simulink model "current_ctl_pi"  (R2023a)
settings: configuration reference "config" (kept outside this file)
model workspace (MAT data in the model file):
  bw = Simulink.Parameter
  bw.Value = 100
  bw.Description = '电流环百分比增益 %  100 表示 100%'
  bw.DataType = 'single'
  bw.Complexity = 'real'
  bw.Dimensions = [1 1]
  dt = Simulink.Parameter
  dt.Value = 5e-05
  dt.Description = '电流环运行频率 用于增益计算'
  dt.DataType = 'single'
  dt.Complexity = 'real'
  dt.Dimensions = [1 1]
  flux = Simulink.Parameter
  flux.Value = 0.0071333
  flux.Description = '磁链系数 Wb'
  flux.DataType = 'single'
  flux.Complexity = 'real'
  flux.Dimensions = [1 1]
  fs = Simulink.Parameter
  fs.Value = 20000
  fs.Description = '电流环运行频率 用于增益计算'
  fs.DataType = 'single'
  fs.Complexity = 'real'
  fs.Dimensions = [1 1]
  kFs = Simulink.Parameter
  kFs.Value = 20000
  kFs.Description = '电流环控制频率 HZ  用于设定模块仿真'
  kFs.DataType = 'double'
  kFs.Complexity = 'real'
  kFs.Dimensions = [1 1]
  ld = Simulink.Parameter
  ld.Value = 0.00059
  ld.Description = '定子电感 H'
  ld.DataType = 'single'
  ld.Complexity = 'real'
  ld.Dimensions = [1 1]
  ld_inv = Simulink.Parameter
  ld_inv.Value = 1694.91525424
  ld_inv.Description = '定子电感 H'
  ld_inv.DataType = 'single'
  ld_inv.Complexity = 'real'
  ld_inv.Dimensions = [1 1]
  lq = Simulink.Parameter
  lq.Value = 0.00059
  lq.Description = '定子电感 H'
  lq.DataType = 'single'
  lq.Complexity = 'real'
  lq.Dimensions = [1 1]
  lq_inv = Simulink.Parameter
  lq_inv.Value = 1694.91525424
  lq_inv.Description = '定子电感 H'
  lq_inv.DataType = 'single'
  lq_inv.Complexity = 'real'
  lq_inv.Dimensions = [1 1]
  r = Simulink.Parameter
  r.Value = 1.02
  r.Description = '定子电阻 ohm'
  r.DataType = 'single'
  r.Complexity = 'real'
  r.Dimensions = [1 1]
libraries: simulink x4, eeTransforms x2
settings Model: DataDictionary=model_config.sldd  ParameterArgumentNames=bw,dt,flux,fs,ld,ld_inv,lq,lq_inv,r  Creator=huangcheng  LastModifiedBy=Administrator
settings ConfigSetRef: SourceName=config

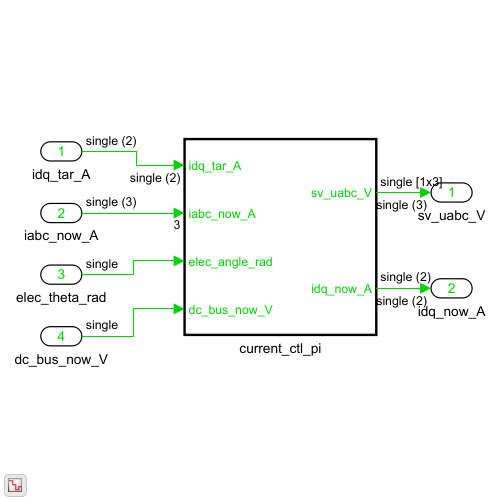
[thumbnail: Simulink's stored preview of the top-level diagram]
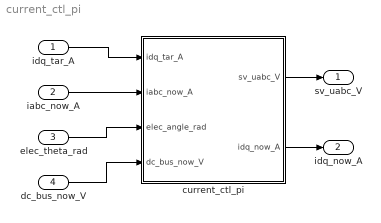
== system current_ctl_pi ==
  idq_tar_A : Inport  OutDataTypeStr=single  PortDimensions=2
  iabc_now_A : Inport  Port=2  OutDataTypeStr=single  PortDimensions=3
  elec_theta_rad : Inport  Port=3  OutDataTypeStr=single  PortDimensions=1
  dc_bus_now_V : Inport  Port=4
  current_ctl_pi : Subsystem  TreatAsAtomicUnit=on  SystemSampleTime=1/kFs
  sv_uabc_V : Outport  OutDataTypeStr=single  PortDimensions=3
  idq_now_A : Outport  Port=2  OutDataTypeStr=single  PortDimensions=2
  wires:
  current_ctl_pi/1(sv_uabc_V) -> sv_uabc_V/1
  idq_tar_A/1 -> current_ctl_pi/1(idq_tar_A)
  elec_theta_rad/1 -> current_ctl_pi/3(elec_angle_rad)
  iabc_now_A/1 -> current_ctl_pi/2(iabc_now_A)
  current_ctl_pi/2(idq_now_A) -> idq_now_A/1
  dc_bus_now_V/1 -> current_ctl_pi/4(dc_bus_now_V)

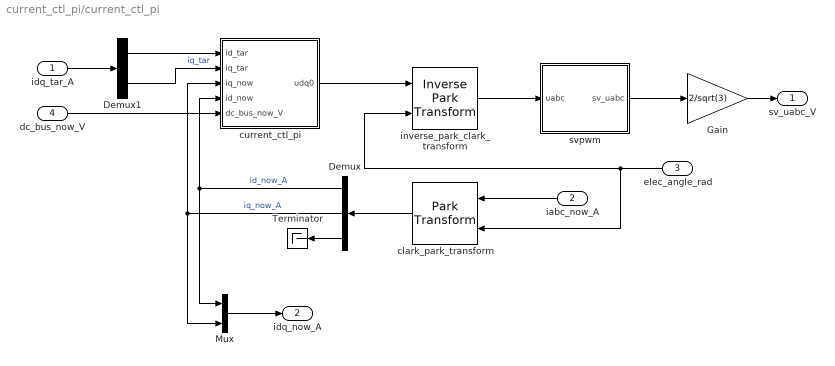
== system current_ctl_pi/current_ctl_pi ==
  idq_tar_A : Inport  OutDataTypeStr=single  PortDimensions=2
  iabc_now_A : Inport  Port=2  PortDimensions=3
  elec_angle_rad : Inport  Port=3
  dc_bus_now_V : Inport  Port=4
  Demux : Demux  Outputs=3
  Demux1 : Demux  Outputs=2
  Gain : Gain  Gain=2/sqrt(3)
  Mux : Mux  Inputs=2
  Terminator : Terminator
  "clark_park_transform " : eeTransforms/Park Transform  AxisAlignment=D-axis  PowerInvariant=off
  current_ctl_pi : Subsystem  SystemSampleTime=5e-5
  inverse_park_clark_transform : eeTransforms/Inverse Park Transform  AxisAlignment=D-axis  PowerInvariant=off
      settings: LibrarySourceBlock=|
      | ee_sl_lib/Mathematical
      | Transforms/Inverse
      | Park Transform
  "svpwm " : MATLAB Function
  sv_uabc_V : Outport
  idq_now_A : Outport  Port=2
  wires:
  "clark_park_transform "/1 -> Demux/1
  Demux/2 -> Mux/2, current_ctl_pi/3(iq_now)  "iq_now_A"
  Demux1/2 -> current_ctl_pi/2(iq_tar)  "iq_tar"
  idq_tar_A/1 -> Demux1/1
  elec_angle_rad/1 -> "clark_park_transform "/2, inverse_park_clark_transform/2
  inverse_park_clark_transform/1 -> "svpwm "/1(uabc)
  current_ctl_pi/1(udq0) -> inverse_park_clark_transform/1
  Demux/1 -> Mux/1, current_ctl_pi/4(id_now)  "id_now_A"
  Demux1/1 -> current_ctl_pi/1(id_tar)
  "svpwm "/1(sv_uabc) -> Gain/1
  iabc_now_A/1 -> "clark_park_transform "/1
  Demux/3 -> Terminator/1
  Mux/1 -> idq_now_A/1
  dc_bus_now_V/1 -> current_ctl_pi/5(dc_bus_now_V)
  Gain/1 -> sv_uabc_V/1

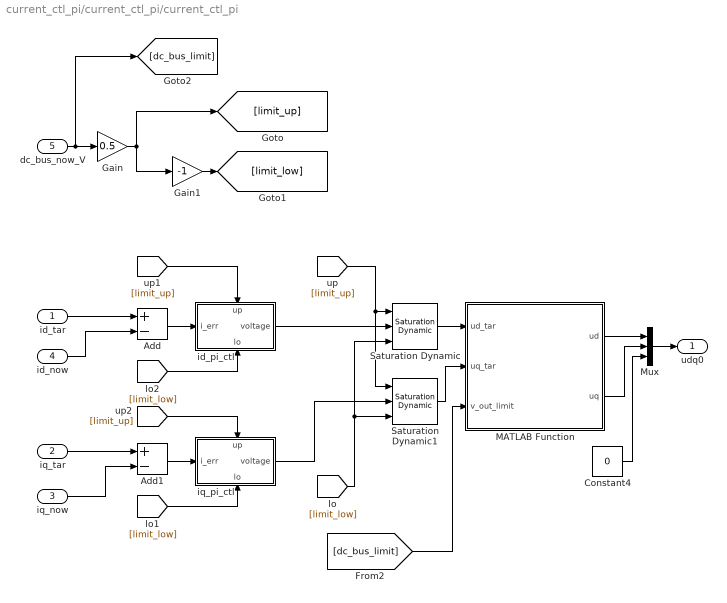
== system current_ctl_pi/current_ctl_pi/current_ctl_pi ==
  id_tar : Inport
  iq_tar : Inport  Port=2
  iq_now : Inport  Port=3
  id_now : Inport  Port=4
  dc_bus_now_V : Inport  Port=5
  Add : Sum  Inputs=+-
  Add1 : Sum  Inputs=+-
  Constant4 : Constant  Value=0  OutDataTypeStr=single
  Gain : Gain  Gain=0.5
  Gain1 : Gain  Gain=-1
  MATLAB Function : MATLAB Function  TreatAsAtomicUnit=on
  Mux : Mux  Inputs=3
  Saturation Dynamic : simulink/Discontinuities/Saturation Dynamic  OutMin=[]  OutMax=[]  OutDataTypeStr=Inherit: Same as second input  OutDataType=fixdt(1, 16)  OutScaling=2^-10  DoSatur=off
  Saturation Dynamic1 : simulink/Discontinuities/Saturation Dynamic  OutMin=[]  OutMax=[]  OutDataTypeStr=Inherit: Same as second input  OutDataType=fixdt(1, 16)  OutScaling=2^-10  DoSatur=off
  id_pi_ctl : Subsystem
      settings: PortSchema="{\"entries\":[{\"content\":{\"sides\":[{\"content\":{\"connectorIds\":[\"In1\"]},\"type\":\"ConnectorPlacement.EquallySpacedRectSide\",\"uuid\":\"c1844c88-1674-45a0-9162-ed878ab5f875\"},{\"content\":{\"connectorIds\":[\"Out1\"],\"side\":\"RIGHT\"},\"type\":\"ConnectorPlacement.EquallySpacedRectSide\",\"uuid\":\"e31a8f95-4a38-441d-8910-e435a2d47625\"},{\"content\":{\"connectorIds\":[\"In2\"],\"side\":\"TOP\"},\"type\":\"ConnectorPlacement.EquallySpacedRectSide\",\"uuid\":\"19790e4f-e49d-4c5f-9b24-5e7784090165\"},{\"content\":{\"connectorIds\":[\"In3\"],\"side\":\"BOTTOM\"},\"type\":\"ConnectorPlacement.EquallySpacedRectSide\",\"uuid\":\"52b1564c-0973-4838-ba98-4979f0071d24\"}]},\"type\":\"ConnectorPlacement.EquallySpacedConnector\",\"uuid\":\"b4def285-36eb-4924-b022-daf3bf206908\"}],\"packageUris\":[\"http://schema.mathworks.com/mf0/Connector/R2020b\"],\"version\":\"1.0\"}"
  iq_pi_ctl : Subsystem
      settings: PortSchema="{\"entries\":[{\"content\":{\"sides\":[{\"content\":{\"connectorIds\":[\"In1\"]},\"type\":\"ConnectorPlacement.EquallySpacedRectSide\",\"uuid\":\"c1844c88-1674-45a0-9162-ed878ab5f875\"},{\"content\":{\"connectorIds\":[\"Out1\"],\"side\":\"RIGHT\"},\"type\":\"ConnectorPlacement.EquallySpacedRectSide\",\"uuid\":\"e31a8f95-4a38-441d-8910-e435a2d47625\"},{\"content\":{\"connectorIds\":[\"In2\"],\"side\":\"TOP\"},\"type\":\"ConnectorPlacement.EquallySpacedRectSide\",\"uuid\":\"19790e4f-e49d-4c5f-9b24-5e7784090165\"},{\"content\":{\"connectorIds\":[\"In3\"],\"side\":\"BOTTOM\"},\"type\":\"ConnectorPlacement.EquallySpacedRectSide\",\"uuid\":\"52b1564c-0973-4838-ba98-4979f0071d24\"}]},\"type\":\"ConnectorPlacement.EquallySpacedConnector\",\"uuid\":\"b4def285-36eb-4924-b022-daf3bf206908\"}],\"packageUris\":[\"http://schema.mathworks.com/mf0/Connector/R2020b\"],\"version\":\"1.0\"}"
  udq0 : Outport  VectorParamsAs1DForOutWhenUnconnected=off
  wires:
  Mux/1 -> udq0/1
  MATLAB Function/2(uq) -> Mux/2
  Constant4/1 -> Mux/3
  MATLAB Function/1(ud) -> Mux/1
  Add/1 -> id_pi_ctl/1(i_err)
  id_tar/1 -> Add/1
  id_now/1 -> Add/2
  iq_tar/1 -> Add1/1
  Add1/1 -> iq_pi_ctl/1(i_err)
  iq_now/1 -> Add1/2
  id_pi_ctl/1(voltage) -> Saturation Dynamic/2
  iq_pi_ctl/1(voltage) -> Saturation Dynamic1/2
  Saturation Dynamic/1 -> MATLAB Function/1(ud_tar)
  Saturation Dynamic1/1 -> MATLAB Function/2(uq_tar)
  [dc_bus_limit] -> MATLAB Function/3(v_out_limit)
  dc_bus_now_V/1 -> [dc_bus_limit], Gain/1
  Gain/1 -> Gain1/1, [limit_up]
  Gain1/1 -> [limit_low]
  [limit_up] -> Saturation Dynamic1/1, Saturation Dynamic/1
  [limit_low] -> Saturation Dynamic1/3, Saturation Dynamic/3
  [limit_low] -> iq_pi_ctl/3(lo)
  [limit_up] -> id_pi_ctl/2(up)
  [limit_up] -> iq_pi_ctl/2(up)
  [limit_low] -> id_pi_ctl/3(lo)

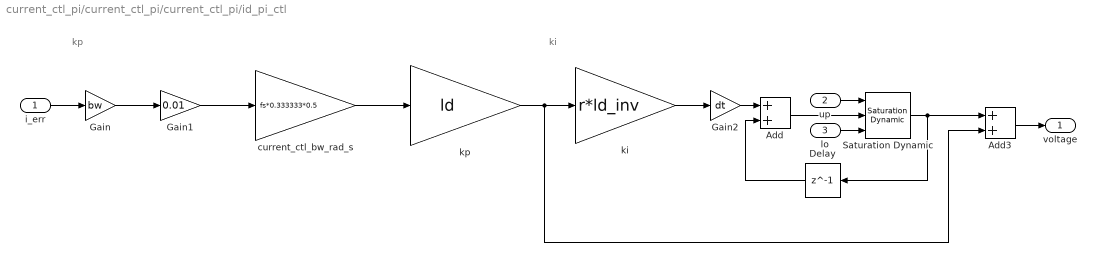
== system current_ctl_pi/current_ctl_pi/current_ctl_pi/id_pi_ctl ==
  note: kp
  note: ki
  i_err : Inport
  up : Inport  Port=2
  lo : Inport  Port=3
  Add : Sum
  Add3 : Sum
  Delay : Delay  DelayLength=1  StateName=id_ki_int
  Gain : Gain  Gain=bw
  Gain1 : Gain  Gain=0.01
  Gain2 : Gain  Gain=dt
  Saturation Dynamic : simulink/Discontinuities/Saturation Dynamic  OutMin=[]  OutMax=[]  OutDataTypeStr=Inherit: Same as second input  OutDataType=fixdt(1, 16)  OutScaling=2^-10  DoSatur=off
  current_ctl_bw_rad_s : Gain  Gain=fs*0.333333*0.5
  ki : Gain  Gain=r*ld_inv
  kp : Gain  Gain=ld
  voltage : Outport
  wires:
  current_ctl_bw_rad_s/1 -> kp/1
  ki/1 -> Gain2/1
  Add3/1 -> voltage/1
  kp/1 -> Add3/2, ki/1
  i_err/1 -> Gain/1
  Gain/1 -> Gain1/1
  Gain1/1 -> current_ctl_bw_rad_s/1
  Saturation Dynamic/1 -> Delay/1, Add3/1
  Gain2/1 -> Add/1
  Delay/1 -> Add/2
  Add/1 -> Saturation Dynamic/2
  up/1 -> Saturation Dynamic/1
  lo/1 -> Saturation Dynamic/3

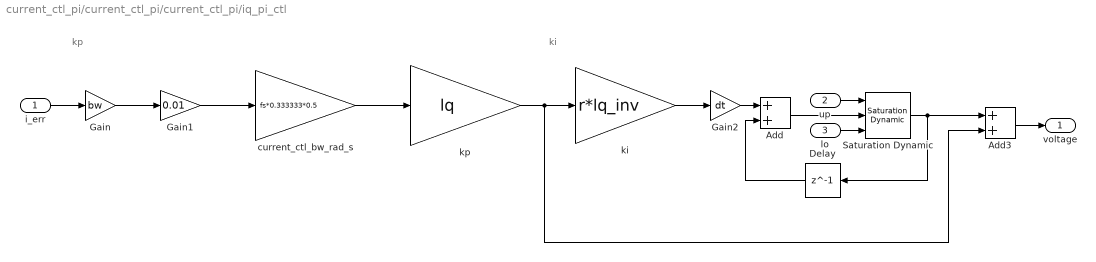
== system current_ctl_pi/current_ctl_pi/current_ctl_pi/iq_pi_ctl ==
  note: ki
  note: kp
  i_err : Inport
  up : Inport  Port=2
  lo : Inport  Port=3
  Add : Sum
  Add3 : Sum
  Delay : Delay  DelayLength=1  StateName=iq_ki_int
  Gain : Gain  Gain=bw
  Gain1 : Gain  Gain=0.01
  Gain2 : Gain  Gain=dt
  Saturation Dynamic : simulink/Discontinuities/Saturation Dynamic  OutMin=[]  OutMax=[]  OutDataTypeStr=Inherit: Same as second input  OutDataType=fixdt(1, 16)  OutScaling=2^-10  DoSatur=off
  current_ctl_bw_rad_s : Gain  Gain=fs*0.333333*0.5
  ki : Gain  Gain=r*lq_inv
  kp : Gain  Gain=lq
  voltage : Outport
  wires:
  lo/1 -> Saturation Dynamic/3
  up/1 -> Saturation Dynamic/1
  Add/1 -> Saturation Dynamic/2
  Delay/1 -> Add/2
  Gain2/1 -> Add/1
  Saturation Dynamic/1 -> Add3/1, Delay/1
  Gain1/1 -> current_ctl_bw_rad_s/1
  Gain/1 -> Gain1/1
  i_err/1 -> Gain/1
  kp/1 -> ki/1, Add3/2
  Add3/1 -> voltage/1
  ki/1 -> Gain2/1
  current_ctl_bw_rad_s/1 -> kp/1

== matlab function current_ctl_pi/current_ctl_pi/MATLAB Function ==
  data: ud_tar input; ud output; uq_tar input; v_out_limit input; uq output
function [ud, uq] = udq_max_lim(ud_tar, uq_tar, v_out_limit)

uq_max = sqrt(v_out_limit^2-ud_tar^2);

if(uq_tar > uq_max)
    uq_tar = uq_max;
elseif(uq_tar < -uq_max)
    uq_tar = -uq_max;    
end
uq = single(uq_tar);
ud = single(ud_tar);

== matlab function current_ctl_pi/svpwm  ==
  data: uabc input; sv_uabc output
function sv_uabc  = svpwm_genrate(uabc)
%最大值最小值法
va = single(uabc(1));
vb = single(uabc(2));
vc = single(uabc(3));
sv_uabc = single(zeros(1,3));

if va>vb
    vmax = va;
    vmin = vb;
else
    vmax = vb;
    vmin = va;
end

if vc>vmax
    vmax = vc;
elseif vc<vmin
    vmin = vc;
end

vcom = 0.5*(vmax+vmin);

ua = va-vcom;
ub = vb-vcom;
uc = vc-vcom;

sv_uabc(1) = single(ua);
sv_uabc(2) = single(ub);
sv_uabc(3) = single(uc);
